simulink model "TesLedsColision"  (R2024b)
settings: Solver=VariableStepAuto  StartTime=0.0  StopTime=inf  RelTol=1e-3
settings Model: Creator=Chenfu  LastModifiedBy=Chenfu

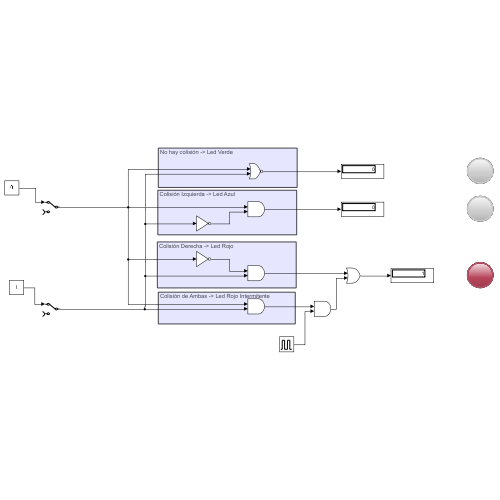
[thumbnail: Simulink's stored preview of the top-level diagram]
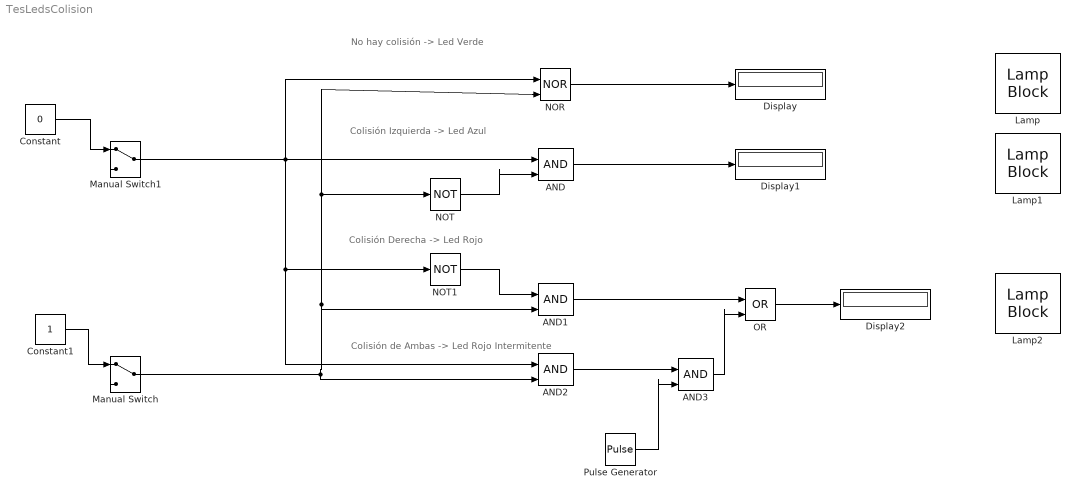
== system TesLedsColision ==
  note: Colisión de Ambas -> Led Rojo Intermitente
  note: No hay colisión -> Led Verde
  note: Colisión Izquierda -> Led Azul
  note: Colisión Derecha -> Led Rojo
  AND{,1..3} (4 alike) : Logic  IconShape=distinctive  AllPortsSameDT=off  OutDataTypeStr=boolean
  Constant : Constant  Value=0
  Constant1 : Constant
  Display : Display
  Display1 : Display
  Display2 : Display
  Lamp : LampBlock  LabelPosition=Hide
  Lamp1 : LampBlock  LabelPosition=Hide
  Lamp2 : LampBlock  LabelPosition=Hide
  Manual Switch : ManualSwitch
  Manual Switch1 : ManualSwitch
  NOR : Logic  Operator=NOR  IconShape=distinctive  AllPortsSameDT=off  OutDataTypeStr=boolean
  NOT : Logic  Operator=NOT  IconShape=distinctive  AllPortsSameDT=off  OutDataTypeStr=boolean
  NOT1 : Logic  Operator=NOT  IconShape=distinctive  AllPortsSameDT=off  OutDataTypeStr=boolean
  OR : Logic  Operator=OR  IconShape=distinctive  AllPortsSameDT=off  OutDataTypeStr=boolean
  Pulse Generator : DiscretePulseGenerator  PulseType=Time based  Period=1  PulseWidth=50
  wires:
  Manual Switch/1 -> AND2/2, NOR/2, NOT/1, AND1/2
  Constant1/1 -> Manual Switch/1
  AND/1 -> Display1/1
  NOR/1 -> Display/1
  Manual Switch1/1 -> NOR/1, AND/1, AND2/1, NOT1/1
  Pulse Generator/1 -> AND3/2
  Constant/1 -> Manual Switch1/1
  OR/1 -> Display2/1
  NOT1/1 -> AND1/1
  AND1/1 -> OR/1
  NOT/1 -> AND/2
  AND3/1 -> OR/2
  AND2/1 -> AND3/1
